simulink model "Q4"  (R2022a)
settings: Solver=FixedStepDiscrete  StartTime=0.0  StopTime=1.0  FixedStep=1  RelTol=1e-3  EnableMultiTasking=on
settings Model: ExtModeTrigDuration=2  Creator=parsa  LastModifiedBy=Parsa Noori
settings OptimizationCC: EnhancedBackFolding=on  PassReuseOutputArgsAs=Individual arguments  ZeroExternalMemoryAtStartup=off  ZeroInternalMemoryAtStartup=off  MaxStackSize=64  OptimizeBlockOrder=speed  DifferentSizesBufferReuse=on  OptimizationCustomize=off  EfficientTunableParamExpr=on
settings DebuggingCC: ParameterTunabilityLossMsg=error
settings HardwareCC: ProdBitPerInt=16  ProdBitPerPointer=16  ProdBitPerSizeT=16  ProdBitPerPtrDiffT=16  ProdLargestAtomicFloat=None  ProdWordSize=8  ProdHWDeviceType=Atmel->AVR
settings ModelReferenceCC: EnableRefExpFcnMdlSchedulingChecks=off
settings SFSimCC: MATLABDynamicMemAlloc=off
settings RTWCC: SystemTargetFile=ert.tlc  HardwareBoard=Arduino Uno  TemplateMakefile=ert_default_tmf  GenerateReport=on  Toolchain=Arduino AVR  BuildConfiguration=Faster Runs  LaunchReport=on  GenerateWebview=on  GenerateCodeMetricsReport=on
settings CodeAppCC: ForceParamTrailComments=on  IgnoreCustomStorageClasses=off  OperatorAnnotations=on  SimulinkDataObjDesc=on  SFDataObjDesc=on  InsertBlockDesc=on
settings ERTTargetCC: SupportContinuousTime=on  SupportVariableSizeSignals=on  ExtModeTransport=3  ExtModeStaticAlloc=on  ExtModeStaticAllocSize=250  ExtModeMexFile=ext_xcp  ExtModeIntrfLevel=Level2 - Open

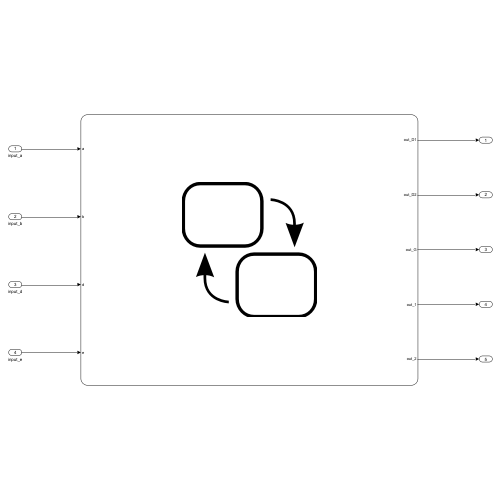
[thumbnail: Simulink's stored preview of the top-level diagram]
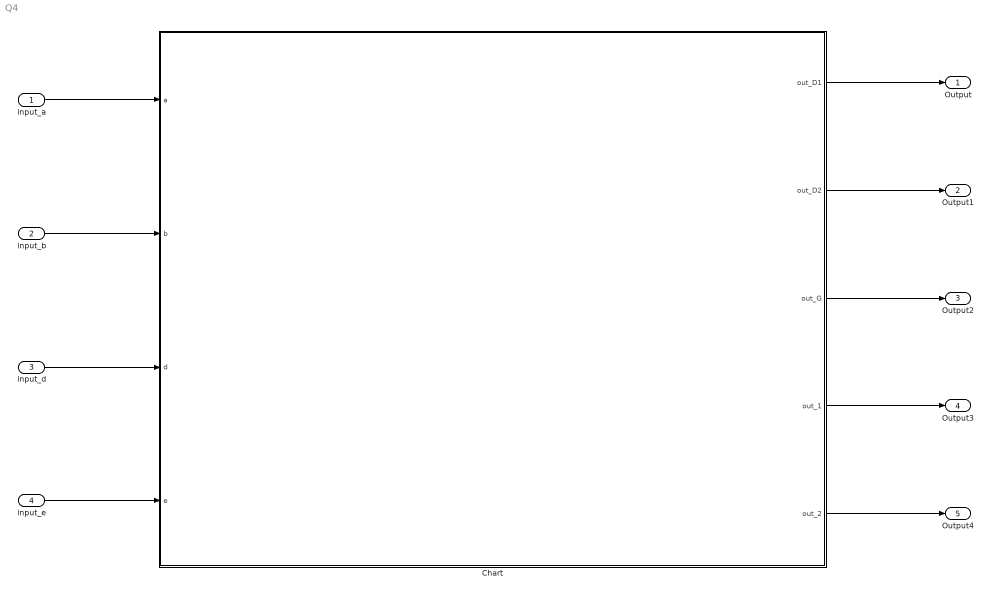
== system Q4 ==
  input_a : Inport
  input_b : Inport  Port=2
  input_d : Inport  Port=3
  input_e : Inport  Port=4
  Chart : Stateflow chart  TreatAsAtomicUnit=on
      settings: PortSchema="{\"entries\":[{\"content\":{\"sides\":[{\"content\":{\"connectorIds\":[\"In4\",\"In3\",\"In1\",\"In2\"]},\"type\":\"ConnectorPlacement.EquallySpacedRectSide\",\"uuid\":\"41448cd1-9580-459b-af44-d3ac9f27b047\"},{\"content\":{\"connectorIds\":[\"Out1\",\"Out2\",\"Out3\",\"Out4\",\"Out5\"],\"side\":\"RIGHT\"},\"type\":\"ConnectorPlacement.EquallySpacedRectSide\",\"uuid\":\"a58346ce-fd7a-400b-9ede-9b1269e92471\"},{\"content\":{\"connectorIds\":[],\"side\":\"TOP\"},\"type\":\"ConnectorPlacement.EquallySpacedRectSide\",\"uuid\":\"077397c2-f73f-4a70-b37c-4d6d98b6329c\"}]},\"type\":\"ConnectorPlacement.EquallySpacedConnector\",\"uuid\":\"b02b47b2-95cd-4f1f-98ff-e8447d9d7227\"}],\"packageUris\":[\"http://schema.mathworks.com/mf0/Connector/R2020b\"],\"version\":\"1.0\"}"
  Output : Outport
  Output1 : Outport  Port=2
  Output2 : Outport  Port=3
  Output3 : Outport  Port=4
  Output4 : Outport  Port=5
  wires:
  Chart/1(out_D1) -> Output/1
  Chart/2(out_D2) -> Output1/1
  Chart/3(out_G) -> Output2/1
  Chart/5(out_2) -> Output4/1
  Chart/4(out_1) -> Output3/1
  input_a/1 -> Chart/4(a)
  input_b/1 -> Chart/3(b)
  input_d/1 -> Chart/1(d)
  input_e/1 -> Chart/2(e)

== stateflow chart Q4/Chart ==
  state A
    state B [parallel]
      settings: executionOrder=1
      state b1
        entry:
        out_1=1;
      state b2
        entry:
        out_2=1;
      (default) -> b1
      b1 -> b2 : [c==1]{out_1=0;}
      b2 -> b1 : [b && in(C.D.D2)]{out_2=0;}
    state C [parallel]
      settings: executionOrder=2
      state D
        state D1
          entry:
          out_D1=1;
        state D2
          entry:
          out_D2=1;
        (default) -> D1
        D1 -> D2 : [e]{out_D1=0;}
        D2 -> D2 : [e]
      state G
        entry:
        out_G=1;
      (default) -> G
      G -> D : [a]{c=1;out_G=0;}
      D -> G : [d]{out_D2=0;out_D1=0;}
  data: d input; e input; b input; a input; out_D1 output; out_D2 output; out_G output; c local =0; out_1 output; out_2 output
